simulink model "sensor_source"  (R2023b)
settings: Solver=FixedStepAuto  StartTime=0.0  StopTime=10.0  RelTol=1e-3
undefined symbols (not defined in the file): f_Baro_Alt, f_GPS, f_IMU, f_Mag, f_Pitot
settings Model: DataDictionary=sensor_datasheet.sldd  Creator=Aniket  LastModifiedBy=Aniket
settings ConfigComp: DVTestSuiteOptimization=Auto  DVDetectOutOfBounds=on  DVModelReferenceHarness=on  DVHarnessSource=Signal Editor  DVRebuildModelRepresentation=IfChangeIsDetected

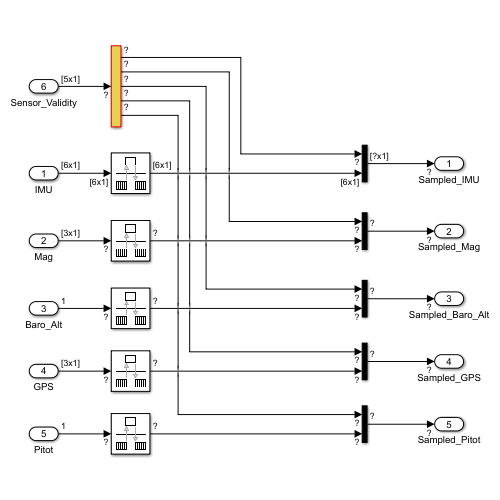
[thumbnail: Simulink's stored preview of the top-level diagram]
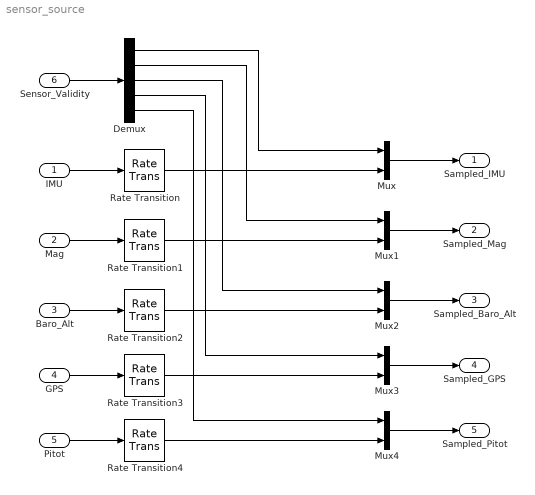
== system sensor_source ==
  IMU : Inport  PortDimensions=[6,1]
  Mag : Inport  Port=2  PortDimensions=[3,1]
  Baro_Alt : Inport  Port=3  PortDimensions=[1]
  GPS : Inport  Port=4  PortDimensions=[3,1]
  Pitot : Inport  Port=5  PortDimensions=[1]
  Sensor_Validity : Inport  Port=6  PortDimensions=[5 1]
  Demux : Demux  Outputs=5
  Mux{,1..4} (5 alike) : Mux  Inputs=2
  Rate Transition : RateTransition  OutPortSampleTime=1/f_IMU
  Rate Transition1 : RateTransition  OutPortSampleTime=1/f_Mag
  Rate Transition2 : RateTransition  OutPortSampleTime=1/f_Baro_Alt
  Rate Transition3 : RateTransition  OutPortSampleTime=1/f_GPS
  Rate Transition4 : RateTransition  OutPortSampleTime=1/f_Pitot
  Sampled_IMU : Outport
  Sampled_Mag : Outport  Port=2
  Sampled_Baro_Alt : Outport  Port=3
  Sampled_GPS : Outport  Port=4
  Sampled_Pitot : Outport  Port=5
  wires:
  Pitot/1 -> Rate Transition4/1
  Mag/1 -> Rate Transition1/1
  Baro_Alt/1 -> Rate Transition2/1
  GPS/1 -> Rate Transition3/1
  IMU/1 -> Rate Transition/1
  Sensor_Validity/1 -> Demux/1
  Rate Transition/1 -> Mux/2
  Mux/1 -> Sampled_IMU/1
  Mux1/1 -> Sampled_Mag/1
  Mux2/1 -> Sampled_Baro_Alt/1
  Mux3/1 -> Sampled_GPS/1
  Mux4/1 -> Sampled_Pitot/1
  Rate Transition1/1 -> Mux1/2
  Rate Transition2/1 -> Mux2/2
  Rate Transition3/1 -> Mux3/2
  Rate Transition4/1 -> Mux4/2
  Demux/1 -> Mux/1
  Demux/2 -> Mux1/1
  Demux/3 -> Mux2/1
  Demux/4 -> Mux3/1
  Demux/5 -> Mux4/1
